simulink model "quadcopter_mdl"  (R2025b)
settings: Solver=VariableStepAuto  StartTime=0.0  StopTime=30  RelTol=1e-3
values from neighbouring files (symbols this model uses):
  A = zeros(12,12)    [lqr_control_euler_mdl.m]
  B = zeros(12,4)    [lqr_control_euler_mdl.m]
  C = zeros(4,12)    [lqr_control_euler_mdl.m]
  G = [0 ; 0; -g]    [quadcopter_params.m]
  gamma = kM/kF    (= 0.0245499181669)    [quadcopter_params.m]
  I = [Ixx 0 0; 0 Iyy 0; 0 0 Izz]    [quadcopter_params.m]
  K = lqr(Ae, Be, Q, R)    [lqr_control_euler_mdl.m]
  kF = 6.11 * 1e-8    (= 6.11e-08)    [quadcopter_params.m]
  L = .5    (= 0.5)    [quadcopter_animate_trajectory.m]    (also in quadcopter_params.m = 0.175)
  m = 0.5    [quadcopter_params.m]
  u0 = [F0; F0; F0; F0]    [lqr_control_euler_mdl.m]
  wi_max = 16000    [quadcopter_params.m]
  x0 = [r0; v0; Theta0; w0]    [lqr_control_euler_mdl.m]
  x1 = [r1; v0; Theta0; w0]    [lqr_control_euler_mdl.m]
undefined symbols (not defined in the file or in its folder): Le
libraries: matrix_library x2, sharedutil x1
settings Model: Creator=Predrag  LastModifiedBy=Predrag

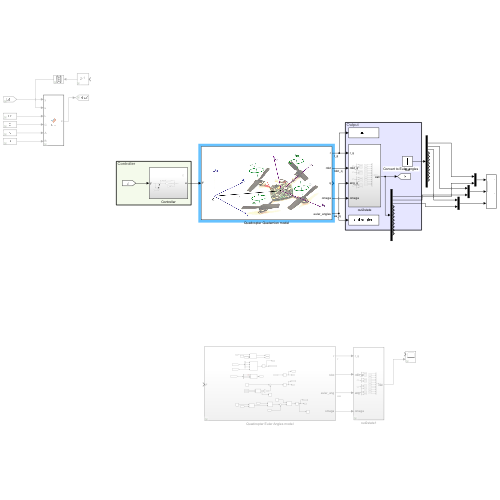
[thumbnail: Simulink's stored preview of the top-level diagram]
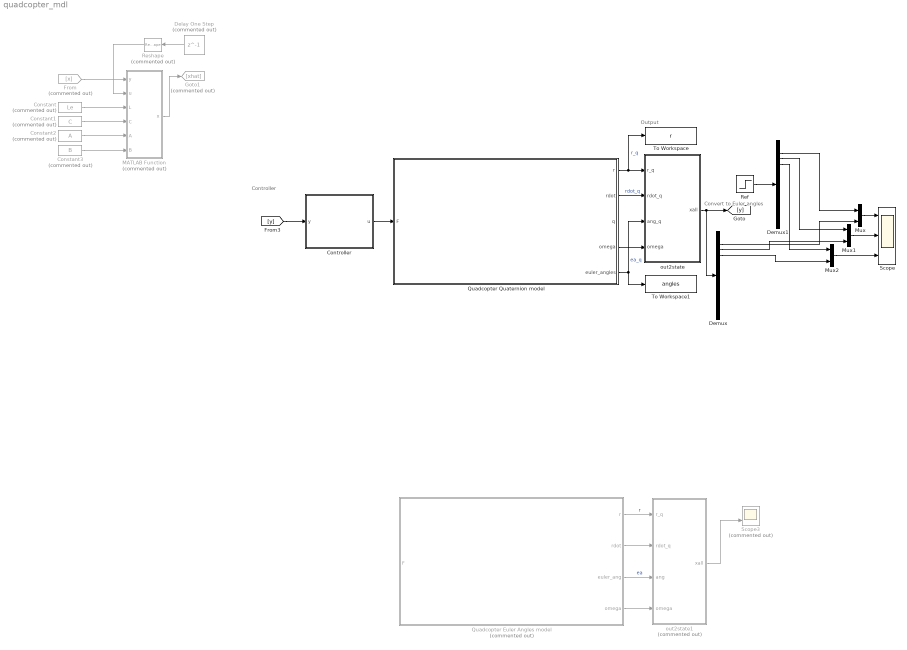
== system quadcopter_mdl ==
  note: Controller
  note: Output
  note: Convert to Euler angles
  Constant : Constant  Commented=on  Value=Le
  Constant1 : Constant  Commented=on  Value=C
  Constant2 : Constant  Commented=on  Value=A
  Constant3 : Constant  Commented=on  Value=B
  Controller : Subsystem
  Delay One Step : Delay  Commented=on  DelayLength=1  InitialCondition=[0;0;0;0]
  Demux : Demux  Outputs=12
  Demux1 : Demux  Outputs=12
  From : From  Commented=on  GotoTag=x
  Goto1 : Goto  Commented=on  GotoTag=xhat
  MATLAB Function : MATLAB Function  Commented=on  TreatAsAtomicUnit=on
  Mux : Mux  Inputs=2
  Mux1 : Mux  Inputs=2
  Mux2 : Mux  Inputs=2
  Quadcopter Euler Angles model : Subsystem  Commented=on
  Quadcopter Quaternion model : Subsystem
      mask Display: image('quadcopter.png');
  Ref : Step  Time=10  Before=x0  After=x1  SampleTime=0
  Reshape : Reshape  Commented=on  OutputDimensionality=Column vector (2-D)
  Scope : Scope  NumInputPorts=3
      settings: ActiveDisplayYMinimum=-0.43277853956601908  ActiveDisplayYMaximum=3.8950068560941729
  Scope3 : Scope  Commented=on  NumInputPorts=2
      settings: ActiveDisplayYMinimum=-4560.5667944463294  ActiveDisplayYMaximum=510.16494144854954  DataLoggingVariableName=ScopeData8
  To Workspace : ToWorkspace  VariableName=r  SaveFormat=Timeseries  SampleTime=-1
  To Workspace1 : ToWorkspace  VariableName=angles  SaveFormat=Timeseries  SampleTime=-1
  out2state : Subsystem
  out2state1 : Subsystem  Commented=on
  wires:
  Controller/1(u) -> Quadcopter Quaternion model/1(F)
  Quadcopter Quaternion model/1(r) -> To Workspace/1, out2state/1(r_q)  "r_q"
  Quadcopter Quaternion model/2(rdot) -> out2state/2(rdot_q)  "rdot_q"
  Quadcopter Quaternion model/4(omega) -> out2state/4(omega)
  MATLAB Function/1(x) -> Goto1/1
  Delay One Step/1 -> Reshape/1
  Constant/1 -> MATLAB Function/3(L)
  Constant1/1 -> MATLAB Function/4(C)
  Constant2/1 -> MATLAB Function/5(A)
  Constant3/1 -> MATLAB Function/6(B)
  Reshape/1 -> MATLAB Function/2(u)
  out2state/1(xall) -> Demux/1, [y]
  From/1 -> MATLAB Function/1(y)
  [y] -> Controller/1(y)
  Quadcopter Euler Angles model/1(r) -> out2state1/1(r_q)  "r"
  Quadcopter Euler Angles model/2(rdot) -> out2state1/2(rdot_q)
  Quadcopter Euler Angles model/3(euler_ang) -> out2state1/3(ang)  "ea"
  Quadcopter Euler Angles model/4(omega) -> out2state1/4(omega)
  out2state1/1(xall) -> Scope3/2
  Quadcopter Quaternion model/5(euler_angles) -> out2state/3(ang_q), To Workspace1/1  "ea_q"
  Ref/1 -> Demux1/1
  Mux/1 -> Scope/1
  Demux1/1 -> Mux/1
  Demux/1 -> Mux/2
  Mux1/1 -> Scope/2
  Demux1/2 -> Mux1/1
  Demux/2 -> Mux1/2
  Mux2/1 -> Scope/3
  Demux1/3 -> Mux2/1
  Demux/3 -> Mux2/2

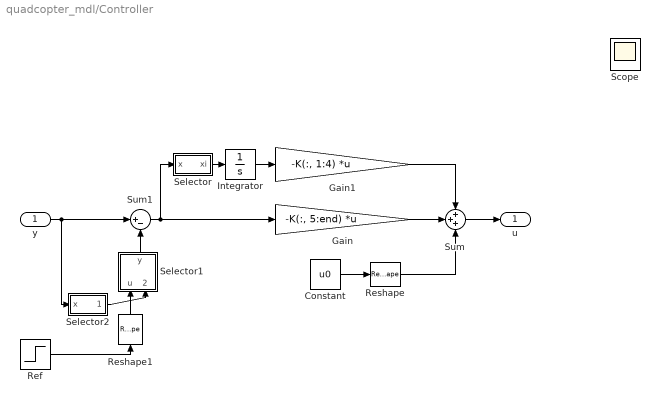
== system quadcopter_mdl/Controller ==
  y : Inport
  Constant : Constant  Value=u0
  Gain : Gain  Gain=-K(:, 5:end)  Multiplication=Matrix(K*u)
  Gain1 : Gain  Gain=-K(:, 1:4)  Multiplication=Matrix(K*u)
  Integrator : Integrator
  Ref : Step  Time=10  Before=x0  After=x1  SampleTime=0
  Reshape : Reshape  OutputDimensionality=Column vector (2-D)
  Reshape1 : Reshape  OutputDimensionality=Column vector (2-D)
  Scope : Scope
      settings: ActiveDisplayYMinimum=-21.181594044209213  ActiveDisplayYMaximum=20.560445182900438  DataLoggingVariableName=ScopeData3
  Selector : MATLAB Function  TreatAsAtomicUnit=on
  Selector1 : MATLAB Function  TreatAsAtomicUnit=on
  Selector2 : MATLAB Function  TreatAsAtomicUnit=on
  Sum : Sum  Inputs=+++
  Sum1 : Sum  Inputs=|+-
  u : Outport
  wires:
  Constant/1 -> Reshape/1
  y/1 -> Selector2/1(x), Sum1/1
  Ref/1 -> Reshape1/1
  Selector/1(xi) -> Integrator/1
  Sum1/1 -> Selector/1(x), Gain/1
  Gain/1 -> Sum/2
  Reshape/1 -> Sum/3
  Sum/1 -> u/1
  Integrator/1 -> Gain1/1
  Gain1/1 -> Sum/1
  Selector1/1(y) -> Sum1/2
  Reshape1/1 -> Selector1/1(u)
  Selector2/1(psi) -> Selector1/2(psi0)

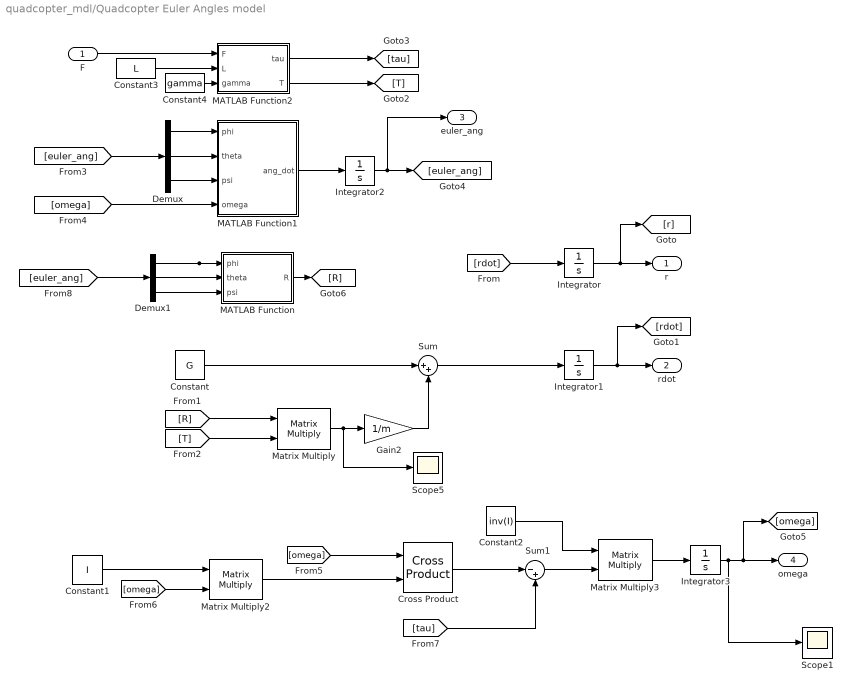
== system quadcopter_mdl/Quadcopter Euler Angles model ==
  F : Inport
  Constant : Constant  Value=G
  Constant1 : Constant  Value=I
  Constant2 : Constant  Value=inv(I)
  Constant3 : Constant  Value=L
  Constant4 : Constant  Value=gamma
  Cross Product : matrix_library/Cross Product
  Demux : Demux  Outputs=3
  Demux1 : Demux  Outputs=3
  Gain2 : Gain  Gain=1/m
  Integrator{,1..3} (4 alike) : Integrator
  MATLAB Function : MATLAB Function  TreatAsAtomicUnit=on
  MATLAB Function1 : MATLAB Function  TreatAsAtomicUnit=on
  MATLAB Function2 : MATLAB Function  TreatAsAtomicUnit=on
  Matrix Multiply : Product  Multiplication=Matrix(*)
  Matrix Multiply2 : Product  Multiplication=Matrix(*)
  Matrix Multiply3 : Product  Multiplication=Matrix(*)
  Scope1 : Scope
      settings: ActiveDisplayYMinimum=-1  ActiveDisplayYMaximum=1
  Scope5 : Scope
      settings: ActiveDisplayYMinimum=-1  ActiveDisplayYMaximum=1  DataLoggingVariableName=ScopeData5
  Sum : Sum  Inputs=|++
  Sum1 : Sum  Inputs=|-+
  r : Outport
  rdot : Outport  Port=2
  euler_ang : Outport  Port=3
  omega : Outport  Port=4
  wires:
  Gain2/1 -> Sum/2
  Matrix Multiply/1 -> Gain2/1, Scope5/1
  MATLAB Function2/1(tau) -> [tau]
  MATLAB Function2/2(T) -> [T]
  Constant4/1 -> MATLAB Function2/3(gamma)
  Constant3/1 -> MATLAB Function2/2(L)
  F/1 -> MATLAB Function2/1(F)
  Constant2/1 -> Matrix Multiply3/1
  Sum1/1 -> Matrix Multiply3/2
  Matrix Multiply3/1 -> Integrator3/1
  [tau] -> Sum1/2
  Constant1/1 -> Matrix Multiply2/1
  [omega] -> Matrix Multiply2/2
  Matrix Multiply2/1 -> Cross Product/2
  [omega] -> Cross Product/1
  Cross Product/1 -> Sum1/1
  Integrator3/1 -> [omega], omega/1, Scope1/1
  [T] -> Matrix Multiply/2
  [R] -> Matrix Multiply/1
  Constant/1 -> Sum/1
  Sum/1 -> Integrator1/1
  [rdot] -> Integrator/1
  Integrator1/1 -> rdot/1, [rdot]
  Integrator/1 -> r/1, [r]
  MATLAB Function1/1(ang_dot) -> Integrator2/1
  Integrator2/1 -> euler_ang/1, [euler_ang]
  Demux/3 -> MATLAB Function1/3(psi)
  Demux/2 -> MATLAB Function1/2(theta)
  Demux/1 -> MATLAB Function1/1(phi)
  [euler_ang] -> Demux/1
  [omega] -> MATLAB Function1/4(omega)
  [euler_ang] -> Demux1/1
  Demux1/1 -> MATLAB Function/1(phi)
  Demux1/2 -> MATLAB Function/2(theta)
  Demux1/3 -> MATLAB Function/3(psi)
  MATLAB Function/1(R) -> [R]

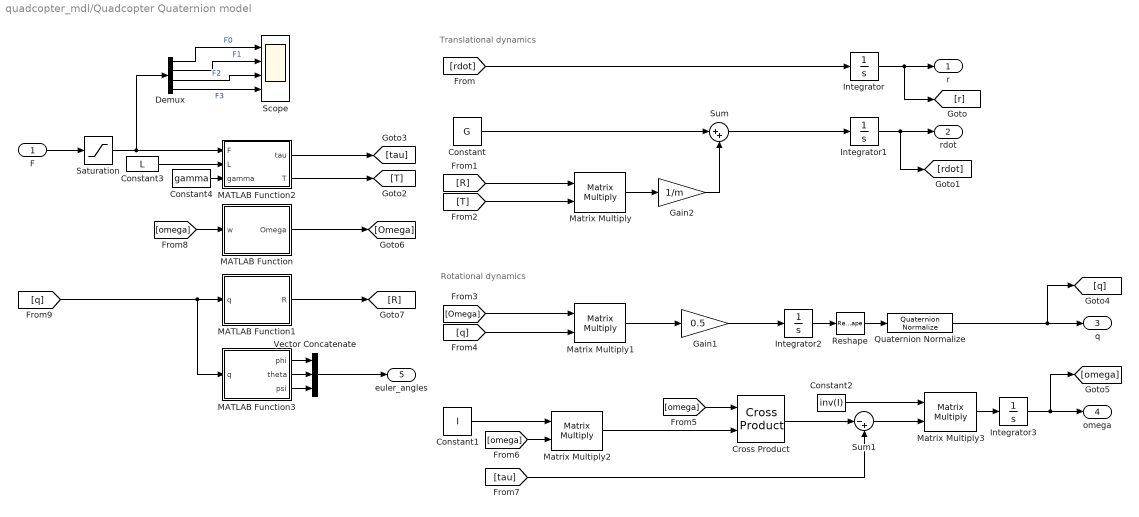
== system quadcopter_mdl/Quadcopter Quaternion model ==
  note: Rotational dynamics
  note: Translational dynamics
  F : Inport
  Constant : Constant  Value=G
  Constant1 : Constant  Value=I
  Constant2 : Constant  Value=inv(I)
  Constant3 : Constant  Value=L
  Constant4 : Constant  Value=gamma
  Cross Product : matrix_library/Cross Product
  Demux : Demux
  Gain1 : Gain  Gain=0.5
  Gain2 : Gain  Gain=1/m
  Integrator : Integrator  InitialCondition=[0; 0; 0]
  Integrator1 : Integrator
  Integrator2 : Integrator  InitialCondition=[1;0;0;0]
  Integrator3 : Integrator
  MATLAB Function : MATLAB Function  TreatAsAtomicUnit=on
  MATLAB Function1 : MATLAB Function  TreatAsAtomicUnit=on
  MATLAB Function2 : MATLAB Function  TreatAsAtomicUnit=on
  MATLAB Function3 : MATLAB Function  TreatAsAtomicUnit=on
  Matrix Multiply{,1..3} (4 alike) : Product  Multiplication=Matrix(*)
  Quaternion Normalize : sharedutil/Quaternion Normalize  aMode=aMode
  Reshape : Reshape  OutputDimensionality=Column vector (2-D)
  Saturation : Saturate  UpperLimit=wi_max^2 * kF  LowerLimit=-wi_max^2 * kF
  Scope : Scope  NumInputPorts=4
      settings: ActiveDisplayYMinimum=0.15058621779069348  ActiveDisplayYMaximum=5.2305717413224651  DataLoggingVariableName=ScopeData2
  Sum : Sum  Inputs=|++
  Sum1 : Sum  Inputs=|-+
  Vector Concatenate : Concatenate  NumInputs=3  Mode=Multidimensional array
  r : Outport
  rdot : Outport  Port=2
  q : Outport  Port=3
  omega : Outport  Port=4
  euler_angles : Outport  Port=5
  wires:
  Integrator/1 -> [r], r/1
  Integrator1/1 -> [rdot], rdot/1
  [rdot] -> Integrator/1
  Sum/1 -> Integrator1/1
  Constant/1 -> Sum/1
  [R] -> Matrix Multiply/1
  [T] -> Matrix Multiply/2
  Integrator2/1 -> Reshape/1
  Gain1/1 -> Integrator2/1
  Matrix Multiply1/1 -> Gain1/1
  [Omega] -> Matrix Multiply1/1
  [q] -> Matrix Multiply1/2
  Integrator3/1 -> omega/1, [omega]
  Cross Product/1 -> Sum1/1
  [omega] -> Cross Product/1
  Matrix Multiply2/1 -> Cross Product/2
  [omega] -> Matrix Multiply2/2
  Constant1/1 -> Matrix Multiply2/1
  [tau] -> Sum1/2
  Matrix Multiply3/1 -> Integrator3/1
  Sum1/1 -> Matrix Multiply3/2
  Constant2/1 -> Matrix Multiply3/1
  [omega] -> MATLAB Function/1(w)
  MATLAB Function/1(Omega) -> [Omega]
  [q] -> MATLAB Function3/1(q), MATLAB Function1/1(q)
  MATLAB Function1/1(R) -> [R]
  Constant3/1 -> MATLAB Function2/2(L)
  Constant4/1 -> MATLAB Function2/3(gamma)
  MATLAB Function2/2(T) -> [T]
  MATLAB Function2/1(tau) -> [tau]
  Matrix Multiply/1 -> Gain2/1
  Gain2/1 -> Sum/2
  Vector Concatenate/1 -> euler_angles/1
  MATLAB Function3/1(phi) -> Vector Concatenate/1
  MATLAB Function3/2(theta) -> Vector Concatenate/2
  MATLAB Function3/3(psi) -> Vector Concatenate/3
  F/1 -> Saturation/1
  Saturation/1 -> Demux/1, MATLAB Function2/1(F)
  Reshape/1 -> Quaternion Normalize/1
  Quaternion Normalize/1 -> [q], q/1
  Demux/2 -> Scope/2  "F1"
  Demux/1 -> Scope/1  "F0"
  Demux/3 -> Scope/3  "F2"
  Demux/4 -> Scope/4  "F3"

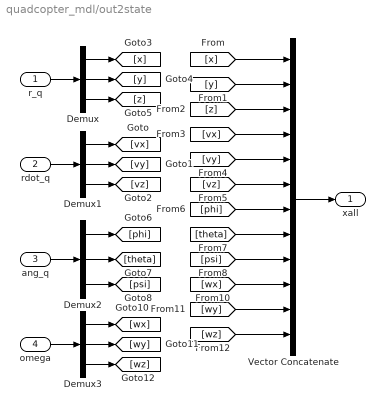
== system quadcopter_mdl/out2state ==
  r_q : Inport
  rdot_q : Inport  Port=2
  ang_q : Inport  Port=3
  omega : Inport  Port=4
  Demux{,1..3} (4 alike) : Demux  Outputs=3
  Vector Concatenate : Concatenate  NumInputs=12  Mode=Multidimensional array
  xall : Outport
  wires:
  r_q/1 -> Demux/1
  rdot_q/1 -> Demux1/1
  Demux1/1 -> [vx]
  Demux1/2 -> [vy]
  Demux1/3 -> [vz]
  Demux/1 -> [x]
  Demux/2 -> [y]
  Demux/3 -> [z]
  [vy] -> Vector Concatenate/5
  [vz] -> Vector Concatenate/6
  [vx] -> Vector Concatenate/4
  [z] -> Vector Concatenate/3
  [y] -> Vector Concatenate/2
  [x] -> Vector Concatenate/1
  ang_q/1 -> Demux2/1
  Demux2/3 -> [psi]
  Demux2/2 -> [theta]
  Demux2/1 -> [phi]
  Demux3/3 -> [wz]
  Demux3/2 -> [wy]
  Demux3/1 -> [wx]
  omega/1 -> Demux3/1
  [phi] -> Vector Concatenate/7
  [theta] -> Vector Concatenate/8
  [psi] -> Vector Concatenate/9
  Vector Concatenate/1 -> xall/1
  [wx] -> Vector Concatenate/10
  [wy] -> Vector Concatenate/11
  [wz] -> Vector Concatenate/12

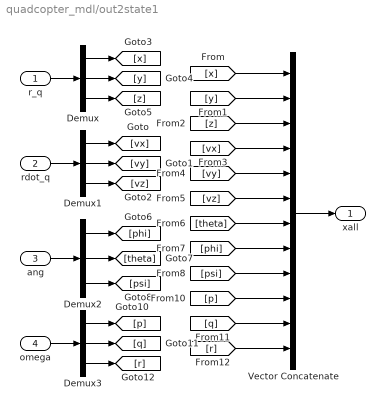
== system quadcopter_mdl/out2state1 ==
  r_q : Inport
  rdot_q : Inport  Port=2
  ang : Inport  Port=3
  omega : Inport  Port=4
  Demux{,1..3} (4 alike) : Demux  Outputs=3
  Vector Concatenate : Concatenate  NumInputs=12  Mode=Multidimensional array
  xall : Outport
  wires:
  Vector Concatenate/1 -> xall/1
  [psi] -> Vector Concatenate/9
  [phi] -> Vector Concatenate/8
  [theta] -> Vector Concatenate/7
  omega/1 -> Demux3/1
  Demux3/1 -> [p]
  Demux3/2 -> [q]
  Demux3/3 -> [r]
  Demux2/1 -> [phi]
  Demux2/2 -> [theta]
  Demux2/3 -> [psi]
  ang/1 -> Demux2/1
  [x] -> Vector Concatenate/1
  [y] -> Vector Concatenate/2
  [z] -> Vector Concatenate/3
  [vx] -> Vector Concatenate/4
  [vz] -> Vector Concatenate/6
  [vy] -> Vector Concatenate/5
  Demux/3 -> [z]
  Demux/2 -> [y]
  Demux/1 -> [x]
  Demux1/3 -> [vz]
  Demux1/2 -> [vy]
  Demux1/1 -> [vx]
  rdot_q/1 -> Demux1/1
  r_q/1 -> Demux/1
  [p] -> Vector Concatenate/10
  [q] -> Vector Concatenate/11
  [r] -> Vector Concatenate/12

== matlab function quadcopter_mdl/Controller/Selector2 ==
  data: x input; psi output
function psi = fcn(x)

psi = x(9);

== matlab function quadcopter_mdl/Quadcopter Quaternion model/MATLAB Function1 ==
  data: q input; R output
function R = fcn(q)

q0 = q(1, 1);
q1 = q(2, 1);
q2 = q(3, 1);
q3 = q(4, 1);


Rx = [q0^2+q1^2-q2^2-q3^2, 2*(q1*q2+q0*q3), 2*(q1*q3 - q0*q2)];
Ry = [2*(q1*q2 - q0*q3), q0^2-q1^2+q2^2-q3^2, 2*(q2*q3 + q0*q1)];
Rz = [2*(q1*q3+q0*q2), 2*(q2*q3 - q0*q1), q0^2-q1^2-q2^2+q3^2];
R_ = [Rx;Ry;Rz];
R = R_';

== matlab function quadcopter_mdl/Quadcopter Quaternion model/MATLAB Function ==
  data: w input; Omega output
function Omega = fcn(w)

wx = w(1);
wy = w(2);
wz = w(3);

Omega = [0, -wx, -wy, -wz; wx, 0, -wz, wy; wy, wz, 0, -wx; wz, -wy, wx, 0];
Omega = [0, -wx, -wy, -wz; wx, 0, wz, -wy; wy, -wz, 0, wx; wz, wy, -wx, 0];

== matlab function quadcopter_mdl/Quadcopter Quaternion model/MATLAB Function2 ==
  data: F input; tau output; L input; gamma input; T output
function [tau, T] = fcn(F, L , gamma)

F1 = F(1);
F2 = F(2);
F3 = F(3);
F4 = F(4);

% Total thrust
T_ = F1 + F2 + F3 + F4;
T = [0; 0; T_];
% Calculate respective torques on each of the axes

tauX = L * (F2 - F4);
tauY = L * (F1 - F3);
tauZ = gamma * (F1 - F2 + F3 - F4);
tau = [tauX;tauY;tauZ];

== matlab function quadcopter_mdl/MATLAB Function ==
  settings: updateMethod=DISCRETE  sampleTime=1e-3
  data: y input; u input; x output; L input; C input; A input; B input
function x = fcn(y, u, L, C, A, B)

persistent yhat;
persistent xhat;

if(isempty(yhat))
    yhat = zeros(7, 1);
end
if(isempty(xhat))
    xhat = zeros(13, 1);
end

xhat = xhat + 6e-3 * (A*xhat + B*u + L * (y - C*xhat));
x = xhat;

== matlab function quadcopter_mdl/Quadcopter Quaternion model/MATLAB Function3 ==
  data: q input; phi output; theta output; psi output
function [phi, theta, psi] = fcn(q)

q0 = q(1, 1);
q1 = q(2, 1);
q2 = q(3, 1);
q3 = q(4, 1);


phi = atan2(2*(q0*q1 +q2*q3), q0^2 - q1^2 - q2^2 + q3^2);
theta = asin(2*(q0*q2 - q3*q1));
psi = atan2(-2*(q0*q3 +q2*q1), q0^2 + q1^2 - q2^2 - q3^2);

== matlab function quadcopter_mdl/Quadcopter Euler Angles model/MATLAB Function ==
  data: phi input; R output; theta input; psi input
function R = fcn(phi, theta, psi)

Rx = [cos(phi) * cos(theta)-sin(phi)*sin(psi)*sin(theta), -cos(phi)*sin(psi), cos(psi)*sin(theta)+cos(theta)*sin(phi)*sin(psi)];
Ry = [cos(theta) * sin(psi)+cos(psi)*sin(phi)*sin(theta), cos(phi)*cos(psi), sin(psi)*sin(theta)-cos(psi)*cos(theta)*sin(phi)];
Rz = [-cos(phi)*sin(theta), sin(phi), cos(phi)*cos(theta)];
R = [Rx;Ry;Rz];

== matlab function quadcopter_mdl/Quadcopter Euler Angles model/MATLAB Function1 ==
  data: phi input; ang_dot output; theta input; psi input; omega input
function ang_dot = fcn(phi, theta, psi, omega)

E = [cos(theta), 0, -cos(phi)*sin(theta); 0 1 sin(phi); sin(theta) 0 cos(phi)*cos(theta)];

ang_dot = inv(E) * omega;

== matlab function quadcopter_mdl/Quadcopter Euler Angles model/MATLAB Function2 ==
  data: F input; tau output; L input; gamma input; T output
function [tau, T] = fcn(F, L , gamma)

F1 = F(1);
F2 = F(2);
F3 = F(3);
F4 = F(4);

% Total thrust
T_ = F1 + F2 + F3 + F4;
T = [0; 0; T_];
% Calculate respective torques on each of the axes

tauX = L * (F2 - F4);
tauY = L * (F1 - F3);
tauZ = gamma * (F1 - F2 + F3 - F4);
tau = [tauX;tauY;tauZ];

== matlab function quadcopter_mdl/Controller/Selector ==
  data: x input; xi output
function xi = fcn(x)

re = x(1:3, 1);
psie = x(9, 1);

xi = [re; psie];

== matlab function quadcopter_mdl/Controller/Selector1 ==
  data: u input; y output; psi0 input
function y = fcn(u, psi0)



u1 = u(1:8);
u2 = u(10:12);
y = [u1; psi0; u2];
